simulink library "Decoders_Lib"  (R2023a)
settings: Solver=ode45  StartTime=0.0  StopTime=10.0  RelTol=1e-3  EnableMultiTasking=on
(part 1 of 2)
settings Model: Creator=uzivatel  LastModifiedBy=Jozko Mrkvicka
settings SolverCC: AlgebraicLoopSolver=TrustRegion
settings DataIOCC: LimitDataPoints=on  SaveFormat=Array  ReturnWorkspaceOutputs=off
settings OptimizationCC: LifeSpan=inf
settings DebuggingCC: UnderspecifiedInitializationDetection=Classic  MergeDetectMultiDrivingBlocksExec=none  SolverPrmCheckMsg=warning  UnconnectedInputMsg=warning  UnconnectedOutputMsg=warning  UnconnectedLineMsg=warning  StateNameClashWarn=warning  SFUnexpectedBacktrackingDiag=warning  SFNoUnconditionalDefaultTransitionDiag=warning  ArithmeticOperatorsInVariantConditions=warning
settings HardwareCC: ProdBitPerPointer=32  ProdBitPerSizeT=32  ProdBitPerPtrDiffT=32  ProdLargestAtomicFloat=None  ProdIntDivRoundTo=Undefined  ProdEndianess=Unspecified  ProdWordSize=32  ProdHWDeviceType=32-bit Generic
settings ModelReferenceCC: EnableRefExpFcnMdlSchedulingChecks=on  PropagateSignalLabelsOutOfModel=off
settings SFSimCC: SimUseLocalCustomCode=off  CustomCodeUndefinedFunction=UseInterfaceOnly
settings RTWCC: RTWUseLocalCustomCode=off
settings CodeAppCC: StateflowObjectComments=on
settings GRTTargetCC: TargetLangStandard=C89/C90 (ANSI)
settings ConfigComp: CovMetricSettings=dw  CovSaveCumulativeToWorkspaceVar=on  CovSaveSingleToWorkspaceVar=on  CovExternalEMLEnable=off

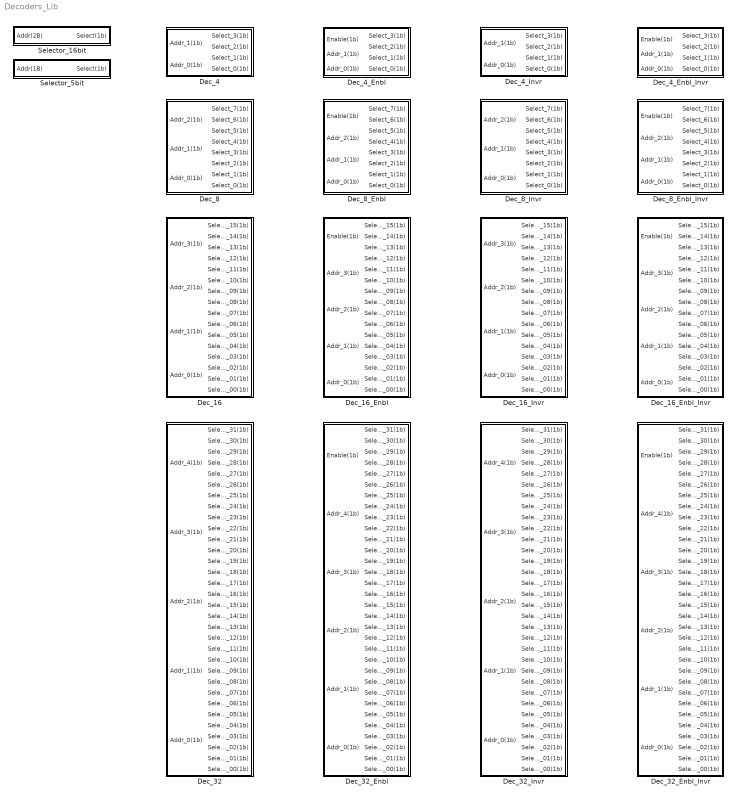
== system Decoders_Lib ==
  Dec_16 : Subsystem  TreatAsAtomicUnit=on
  Dec_16_Enbl : Subsystem  TreatAsAtomicUnit=on
  Dec_16_Enbl_Invr : Subsystem  TreatAsAtomicUnit=on
  Dec_16_Invr : Subsystem  TreatAsAtomicUnit=on
  Dec_32 : Subsystem  TreatAsAtomicUnit=on
  Dec_32_Enbl : Subsystem  TreatAsAtomicUnit=on
  Dec_32_Enbl_Invr : Subsystem  TreatAsAtomicUnit=on
  Dec_32_Invr : Subsystem  TreatAsAtomicUnit=on
  Dec_4 : Subsystem  TreatAsAtomicUnit=on
  Dec_4_Enbl : Subsystem  TreatAsAtomicUnit=on
  Dec_4_Enbl_Invr : Subsystem  TreatAsAtomicUnit=on
  Dec_4_Invr : Subsystem  TreatAsAtomicUnit=on
  Dec_8 : Subsystem  TreatAsAtomicUnit=on
  Dec_8_Enbl : Subsystem  TreatAsAtomicUnit=on
  Dec_8_Enbl_Invr : Subsystem  TreatAsAtomicUnit=on
  Dec_8_Invr : Subsystem  TreatAsAtomicUnit=on
  Selector_16bit : Subsystem
  Selector_5bit : Subsystem

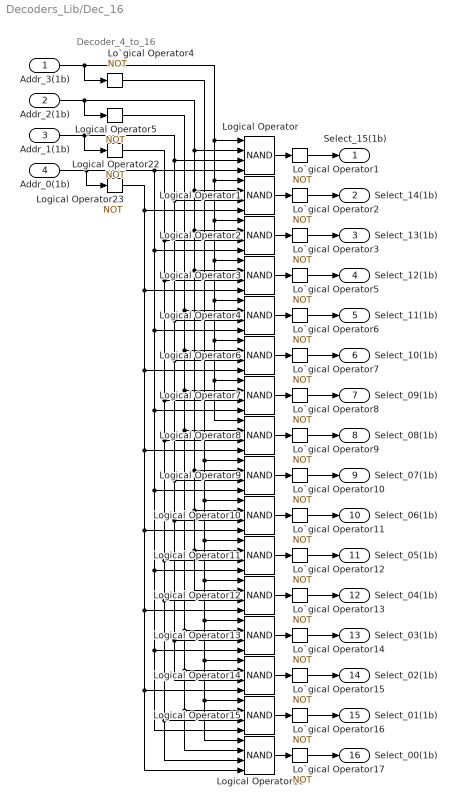
== system Decoders_Lib/Dec_16 ==
  note: Decoder_4_to_16
  Addr_3(1b) : Inport
  Addr_2(1b) : Inport  Port=2
  Addr_1(1b) : Inport  Port=3
  Addr_0(1b) : Inport  Port=4
  Lo`gical Operator{1..17} (17 alike) : Logic  Operator=NOT  IconShape=distinctive  AllPortsSameDT=off  OutDataTypeStr=boolean
  Logical Operator{,1..4,6..16} (16 alike) : Logic  Operator=NAND  Inputs=4  IconShape=distinctive  AllPortsSameDT=off  OutDataTypeStr=boolean
  Logical Operator22 : Logic  Operator=NOT  IconShape=distinctive  AllPortsSameDT=off  OutDataTypeStr=boolean
  Logical Operator23 : Logic  Operator=NOT  IconShape=distinctive  AllPortsSameDT=off  OutDataTypeStr=boolean
  Logical Operator5 : Logic  Operator=NOT  IconShape=distinctive  AllPortsSameDT=off  OutDataTypeStr=boolean
  Select_15(1b) : Outport
  Select_14(1b) : Outport  Port=2
  Select_13(1b) : Outport  Port=3
  Select_12(1b) : Outport  Port=4
  Select_11(1b) : Outport  Port=5
  Select_10(1b) : Outport  Port=6
  Select_09(1b) : Outport  Port=7
  Select_08(1b) : Outport  Port=8
  Select_07(1b) : Outport  Port=9
  Select_06(1b) : Outport  Port=10
  Select_05(1b) : Outport  Port=11
  Select_04(1b) : Outport  Port=12
  Select_03(1b) : Outport  Port=13
  Select_02(1b) : Outport  Port=14
  Select_01(1b) : Outport  Port=15
  Select_00(1b) : Outport  Port=16
  wires:
  Logical Operator22/1 -> Logical Operator2/3, Logical Operator3/3, Logical Operator15/3, Logical Operator16/3, Logical Operator12/3, Logical Operator11/3, Logical Operator8/3, Logical Operator7/3
  Addr_0(1b)/1 -> Logical Operator23/1, Logical Operator/4, Logical Operator9/4, Logical Operator11/4, Logical Operator15/4, Logical Operator13/4, Logical Operator7/4, Logical Operator4/4, Logical Operator2/4
  Logical Operator23/1 -> Logical Operator1/4, Logical Operator16/4, Logical Operator14/4, Logical Operator12/4, Logical Operator10/4, Logical Operator8/4, Logical Operator6/4, Logical Operator3/4
  Logical Operator5/1 -> Logical Operator16/2, Logical Operator15/2, Logical Operator14/2, Logical Operator13/2, Logical Operator8/2, Logical Operator7/2, Logical Operator6/2, Logical Operator4/2
  Addr_3(1b)/1 -> Lo`gical Operator4/1, Logical Operator8/1, Logical Operator7/1, Logical Operator6/1, Logical Operator4/1, Logical Operator3/1, Logical Operator2/1, Logical Operator1/1, Logical Operator/1
  Addr_1(1b)/1 -> Logical Operator22/1, Logical Operator14/3, Logical Operator13/3, Logical Operator10/3, Logical Operator9/3, Logical Operator6/3, Logical Operator4/3, Logical Operator1/3, Logical Operator/3
  Addr_2(1b)/1 -> Logical Operator5/1, Logical Operator3/2, Logical Operator9/2, Logical Operator12/2, Logical Operator11/2, Logical Operator10/2, Logical Operator2/2, Logical Operator1/2, Logical Operator/2
  Lo`gical Operator4/1 -> Logical Operator16/1, Logical Operator15/1, Logical Operator14/1, Logical Operator13/1, Logical Operator12/1, Logical Operator11/1, Logical Operator10/1, Logical Operator9/1
  Logical Operator16/1 -> Lo`gical Operator17/1
  Logical Operator15/1 -> Lo`gical Operator16/1
  Logical Operator14/1 -> Lo`gical Operator15/1
  Logical Operator13/1 -> Lo`gical Operator14/1
  Logical Operator12/1 -> Lo`gical Operator13/1
  Logical Operator11/1 -> Lo`gical Operator12/1
  Logical Operator10/1 -> Lo`gical Operator11/1
  Logical Operator9/1 -> Lo`gical Operator10/1
  Logical Operator8/1 -> Lo`gical Operator9/1
  Logical Operator7/1 -> Lo`gical Operator8/1
  Logical Operator6/1 -> Lo`gical Operator7/1
  Logical Operator4/1 -> Lo`gical Operator6/1
  Logical Operator1/1 -> Lo`gical Operator2/1
  Logical Operator2/1 -> Lo`gical Operator3/1
  Logical Operator3/1 -> Lo`gical Operator5/1
  Logical Operator/1 -> Lo`gical Operator1/1
  Lo`gical Operator1/1 -> Select_15(1b)/1
  Lo`gical Operator2/1 -> Select_14(1b)/1
  Lo`gical Operator3/1 -> Select_13(1b)/1
  Lo`gical Operator5/1 -> Select_12(1b)/1
  Lo`gical Operator6/1 -> Select_11(1b)/1
  Lo`gical Operator7/1 -> Select_10(1b)/1
  Lo`gical Operator8/1 -> Select_09(1b)/1
  Lo`gical Operator9/1 -> Select_08(1b)/1
  Lo`gical Operator10/1 -> Select_07(1b)/1
  Lo`gical Operator11/1 -> Select_06(1b)/1
  Lo`gical Operator12/1 -> Select_05(1b)/1
  Lo`gical Operator13/1 -> Select_04(1b)/1
  Lo`gical Operator14/1 -> Select_03(1b)/1
  Lo`gical Operator15/1 -> Select_02(1b)/1
  Lo`gical Operator16/1 -> Select_01(1b)/1
  Lo`gical Operator17/1 -> Select_00(1b)/1

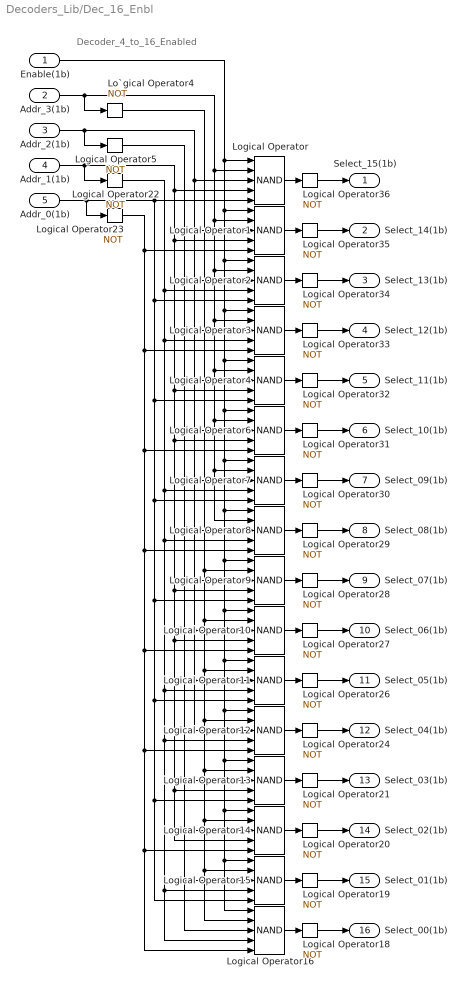
== system Decoders_Lib/Dec_16_Enbl ==
  note: Decoder_4_to_16_Enabled
  Enable(1b) : Inport
  Addr_3(1b) : Inport  Port=2
  Addr_2(1b) : Inport  Port=3
  Addr_1(1b) : Inport  Port=4
  Addr_0(1b) : Inport  Port=5
  Lo`gical Operator4 : Logic  Operator=NOT  IconShape=distinctive  AllPortsSameDT=off  OutDataTypeStr=boolean
  Logical Operator{,1..4,6..16} (16 alike) : Logic  Operator=NAND  Inputs=5  IconShape=distinctive  AllPortsSameDT=off  OutDataTypeStr=boolean
  Logical Operator{5,18..24,26..36} (19 alike) : Logic  Operator=NOT  IconShape=distinctive  AllPortsSameDT=off  OutDataTypeStr=boolean
  Select_15(1b) : Outport
  Select_14(1b) : Outport  Port=2
  Select_13(1b) : Outport  Port=3
  Select_12(1b) : Outport  Port=4
  Select_11(1b) : Outport  Port=5
  Select_10(1b) : Outport  Port=6
  Select_09(1b) : Outport  Port=7
  Select_08(1b) : Outport  Port=8
  Select_07(1b) : Outport  Port=9
  Select_06(1b) : Outport  Port=10
  Select_05(1b) : Outport  Port=11
  Select_04(1b) : Outport  Port=12
  Select_03(1b) : Outport  Port=13
  Select_02(1b) : Outport  Port=14
  Select_01(1b) : Outport  Port=15
  Select_00(1b) : Outport  Port=16
  wires:
  Logical Operator22/1 -> Logical Operator2/4, Logical Operator3/4, Logical Operator7/4, Logical Operator8/4, Logical Operator11/4, Logical Operator12/4, Logical Operator15/4, Logical Operator16/4
  Addr_0(1b)/1 -> Logical Operator/5, Logical Operator2/5, Logical Operator4/5, Logical Operator7/5, Logical Operator9/5, Logical Operator11/5, Logical Operator13/5, Logical Operator15/5, Logical Operator23/1
  Logical Operator23/1 -> Logical Operator1/5, Logical Operator3/5, Logical Operator6/5, Logical Operator8/5, Logical Operator10/5, Logical Operator12/5, Logical Operator14/5, Logical Operator16/5
  Logical Operator5/1 -> Logical Operator4/3, Logical Operator6/3, Logical Operator7/3, Logical Operator8/3, Logical Operator13/3, Logical Operator14/3, Logical Operator15/3, Logical Operator16/3
  Addr_3(1b)/1 -> Logical Operator/2, Logical Operator1/2, Logical Operator2/2, Logical Operator3/2, Logical Operator4/2, Logical Operator6/2, Logical Operator7/2, Logical Operator8/2, Lo`gical Operator4/1
  Addr_1(1b)/1 -> Logical Operator/4, Logical Operator1/4, Logical Operator4/4, Logical Operator6/4, Logical Operator9/4, Logical Operator10/4, Logical Operator13/4, Logical Operator14/4, Logical Operator22/1
  Addr_2(1b)/1 -> Logical Operator/3, Logical Operator1/3, Logical Operator2/3, Logical Operator3/3, Logical Operator9/3, Logical Operator10/3, Logical Operator11/3, Logical Operator12/3, Logical Operator5/1
  Lo`gical Operator4/1 -> Logical Operator9/2, Logical Operator10/2, Logical Operator11/2, Logical Operator12/2, Logical Operator13/2, Logical Operator14/2, Logical Operator15/2, Logical Operator16/2
  Logical Operator16/1 -> Logical Operator18/1
  Logical Operator15/1 -> Logical Operator19/1
  Logical Operator14/1 -> Logical Operator20/1
  Logical Operator13/1 -> Logical Operator21/1
  Logical Operator12/1 -> Logical Operator24/1
  Logical Operator11/1 -> Logical Operator26/1
  Logical Operator10/1 -> Logical Operator27/1
  Logical Operator9/1 -> Logical Operator28/1
  Logical Operator8/1 -> Logical Operator29/1
  Logical Operator7/1 -> Logical Operator30/1
  Logical Operator6/1 -> Logical Operator31/1
  Logical Operator4/1 -> Logical Operator32/1
  Logical Operator1/1 -> Logical Operator35/1
  Logical Operator2/1 -> Logical Operator34/1
  Logical Operator3/1 -> Logical Operator33/1
  Logical Operator/1 -> Logical Operator36/1
  Enable(1b)/1 -> Logical Operator/1, Logical Operator1/1, Logical Operator2/1, Logical Operator3/1, Logical Operator4/1, Logical Operator6/1, Logical Operator7/1, Logical Operator8/1, Logical Operator9/1, Logical Operator10/1, Logical Operator11/1, Logical Operator12/1, Logical Operator13/1, Logical Operator14/1, Logical Operator15/1, Logical Operator16/1
  Logical Operator18/1 -> Select_00(1b)/1
  Logical Operator19/1 -> Select_01(1b)/1
  Logical Operator20/1 -> Select_02(1b)/1
  Logical Operator21/1 -> Select_03(1b)/1
  Logical Operator24/1 -> Select_04(1b)/1
  Logical Operator26/1 -> Select_05(1b)/1
  Logical Operator27/1 -> Select_06(1b)/1
  Logical Operator28/1 -> Select_07(1b)/1
  Logical Operator29/1 -> Select_08(1b)/1
  Logical Operator30/1 -> Select_09(1b)/1
  Logical Operator31/1 -> Select_10(1b)/1
  Logical Operator32/1 -> Select_11(1b)/1
  Logical Operator33/1 -> Select_12(1b)/1
  Logical Operator34/1 -> Select_13(1b)/1
  Logical Operator35/1 -> Select_14(1b)/1
  Logical Operator36/1 -> Select_15(1b)/1

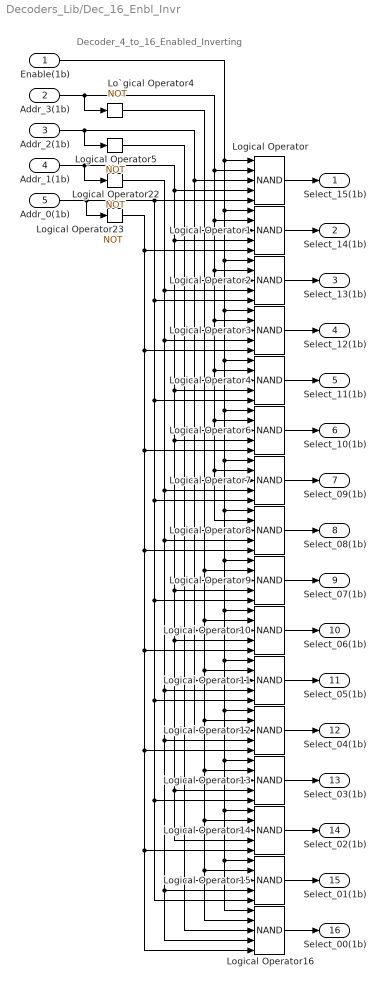
== system Decoders_Lib/Dec_16_Enbl_Invr ==
  note: Decoder_4_to_16_Enabled_Inverting
  Enable(1b) : Inport
  Addr_3(1b) : Inport  Port=2
  Addr_2(1b) : Inport  Port=3
  Addr_1(1b) : Inport  Port=4
  Addr_0(1b) : Inport  Port=5
  Lo`gical Operator4 : Logic  Operator=NOT  IconShape=distinctive  AllPortsSameDT=off  OutDataTypeStr=boolean
  Logical Operator{,1..4,6..16} (16 alike) : Logic  Operator=NAND  Inputs=5  IconShape=distinctive  AllPortsSameDT=off  OutDataTypeStr=boolean
  Logical Operator22 : Logic  Operator=NOT  IconShape=distinctive  AllPortsSameDT=off  OutDataTypeStr=boolean
  Logical Operator23 : Logic  Operator=NOT  IconShape=distinctive  AllPortsSameDT=off  OutDataTypeStr=boolean
  Logical Operator5 : Logic  Operator=NOT  IconShape=distinctive  AllPortsSameDT=off  OutDataTypeStr=boolean
  Select_15(1b) : Outport
  Select_14(1b) : Outport  Port=2
  Select_13(1b) : Outport  Port=3
  Select_12(1b) : Outport  Port=4
  Select_11(1b) : Outport  Port=5
  Select_10(1b) : Outport  Port=6
  Select_09(1b) : Outport  Port=7
  Select_08(1b) : Outport  Port=8
  Select_07(1b) : Outport  Port=9
  Select_06(1b) : Outport  Port=10
  Select_05(1b) : Outport  Port=11
  Select_04(1b) : Outport  Port=12
  Select_03(1b) : Outport  Port=13
  Select_02(1b) : Outport  Port=14
  Select_01(1b) : Outport  Port=15
  Select_00(1b) : Outport  Port=16
  wires:
  Logical Operator22/1 -> Logical Operator2/4, Logical Operator3/4, Logical Operator7/4, Logical Operator8/4, Logical Operator11/4, Logical Operator12/4, Logical Operator15/4, Logical Operator16/4
  Addr_0(1b)/1 -> Logical Operator/5, Logical Operator2/5, Logical Operator4/5, Logical Operator7/5, Logical Operator9/5, Logical Operator11/5, Logical Operator13/5, Logical Operator15/5, Logical Operator23/1
  Logical Operator23/1 -> Logical Operator1/5, Logical Operator3/5, Logical Operator6/5, Logical Operator8/5, Logical Operator10/5, Logical Operator12/5, Logical Operator14/5, Logical Operator16/5
  Logical Operator5/1 -> Logical Operator4/3, Logical Operator6/3, Logical Operator7/3, Logical Operator8/3, Logical Operator13/3, Logical Operator14/3, Logical Operator15/3, Logical Operator16/3
  Addr_3(1b)/1 -> Logical Operator/2, Logical Operator1/2, Logical Operator2/2, Logical Operator3/2, Logical Operator4/2, Logical Operator6/2, Logical Operator7/2, Logical Operator8/2, Lo`gical Operator4/1
  Addr_1(1b)/1 -> Logical Operator/4, Logical Operator1/4, Logical Operator4/4, Logical Operator6/4, Logical Operator9/4, Logical Operator10/4, Logical Operator13/4, Logical Operator14/4, Logical Operator22/1
  Addr_2(1b)/1 -> Logical Operator/3, Logical Operator1/3, Logical Operator2/3, Logical Operator3/3, Logical Operator9/3, Logical Operator10/3, Logical Operator11/3, Logical Operator12/3, Logical Operator5/1
  Lo`gical Operator4/1 -> Logical Operator9/2, Logical Operator10/2, Logical Operator11/2, Logical Operator12/2, Logical Operator13/2, Logical Operator14/2, Logical Operator15/2, Logical Operator16/2
  Logical Operator16/1 -> Select_00(1b)/1
  Logical Operator15/1 -> Select_01(1b)/1
  Logical Operator14/1 -> Select_02(1b)/1
  Logical Operator13/1 -> Select_03(1b)/1
  Logical Operator12/1 -> Select_04(1b)/1
  Logical Operator11/1 -> Select_05(1b)/1
  Logical Operator10/1 -> Select_06(1b)/1
  Logical Operator9/1 -> Select_07(1b)/1
  Logical Operator8/1 -> Select_08(1b)/1
  Logical Operator7/1 -> Select_09(1b)/1
  Logical Operator6/1 -> Select_10(1b)/1
  Logical Operator4/1 -> Select_11(1b)/1
  Logical Operator1/1 -> Select_14(1b)/1
  Logical Operator2/1 -> Select_13(1b)/1
  Logical Operator3/1 -> Select_12(1b)/1
  Logical Operator/1 -> Select_15(1b)/1
  Enable(1b)/1 -> Logical Operator/1, Logical Operator1/1, Logical Operator2/1, Logical Operator3/1, Logical Operator4/1, Logical Operator6/1, Logical Operator7/1, Logical Operator8/1, Logical Operator9/1, Logical Operator10/1, Logical Operator11/1, Logical Operator12/1, Logical Operator13/1, Logical Operator14/1, Logical Operator15/1, Logical Operator16/1

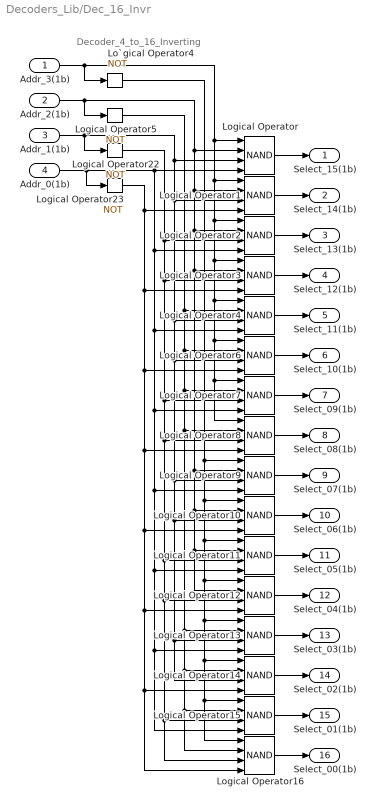
== system Decoders_Lib/Dec_16_Invr ==
  note: Decoder_4_to_16_Inverting
  Addr_3(1b) : Inport
  Addr_2(1b) : Inport  Port=2
  Addr_1(1b) : Inport  Port=3
  Addr_0(1b) : Inport  Port=4
  Lo`gical Operator4 : Logic  Operator=NOT  IconShape=distinctive  AllPortsSameDT=off  OutDataTypeStr=boolean
  Logical Operator{,1..4,6..16} (16 alike) : Logic  Operator=NAND  Inputs=4  IconShape=distinctive  AllPortsSameDT=off  OutDataTypeStr=boolean
  Logical Operator22 : Logic  Operator=NOT  IconShape=distinctive  AllPortsSameDT=off  OutDataTypeStr=boolean
  Logical Operator23 : Logic  Operator=NOT  IconShape=distinctive  AllPortsSameDT=off  OutDataTypeStr=boolean
  Logical Operator5 : Logic  Operator=NOT  IconShape=distinctive  AllPortsSameDT=off  OutDataTypeStr=boolean
  Select_15(1b) : Outport
  Select_14(1b) : Outport  Port=2
  Select_13(1b) : Outport  Port=3
  Select_12(1b) : Outport  Port=4
  Select_11(1b) : Outport  Port=5
  Select_10(1b) : Outport  Port=6
  Select_09(1b) : Outport  Port=7
  Select_08(1b) : Outport  Port=8
  Select_07(1b) : Outport  Port=9
  Select_06(1b) : Outport  Port=10
  Select_05(1b) : Outport  Port=11
  Select_04(1b) : Outport  Port=12
  Select_03(1b) : Outport  Port=13
  Select_02(1b) : Outport  Port=14
  Select_01(1b) : Outport  Port=15
  Select_00(1b) : Outport  Port=16
  wires:
  Logical Operator22/1 -> Logical Operator2/3, Logical Operator3/3, Logical Operator15/3, Logical Operator16/3, Logical Operator12/3, Logical Operator11/3, Logical Operator8/3, Logical Operator7/3
  Addr_0(1b)/1 -> Logical Operator23/1, Logical Operator/4, Logical Operator9/4, Logical Operator11/4, Logical Operator15/4, Logical Operator13/4, Logical Operator7/4, Logical Operator4/4, Logical Operator2/4
  Logical Operator23/1 -> Logical Operator1/4, Logical Operator16/4, Logical Operator14/4, Logical Operator12/4, Logical Operator10/4, Logical Operator8/4, Logical Operator6/4, Logical Operator3/4
  Logical Operator5/1 -> Logical Operator16/2, Logical Operator15/2, Logical Operator14/2, Logical Operator13/2, Logical Operator8/2, Logical Operator7/2, Logical Operator6/2, Logical Operator4/2
  Addr_3(1b)/1 -> Lo`gical Operator4/1, Logical Operator8/1, Logical Operator7/1, Logical Operator6/1, Logical Operator4/1, Logical Operator3/1, Logical Operator2/1, Logical Operator1/1, Logical Operator/1
  Addr_1(1b)/1 -> Logical Operator22/1, Logical Operator14/3, Logical Operator13/3, Logical Operator10/3, Logical Operator9/3, Logical Operator6/3, Logical Operator4/3, Logical Operator1/3, Logical Operator/3
  Addr_2(1b)/1 -> Logical Operator5/1, Logical Operator3/2, Logical Operator9/2, Logical Operator12/2, Logical Operator11/2, Logical Operator10/2, Logical Operator2/2, Logical Operator1/2, Logical Operator/2
  Lo`gical Operator4/1 -> Logical Operator16/1, Logical Operator15/1, Logical Operator14/1, Logical Operator13/1, Logical Operator12/1, Logical Operator11/1, Logical Operator10/1, Logical Operator9/1
  Logical Operator16/1 -> Select_00(1b)/1
  Logical Operator15/1 -> Select_01(1b)/1
  Logical Operator14/1 -> Select_02(1b)/1
  Logical Operator13/1 -> Select_03(1b)/1
  Logical Operator12/1 -> Select_04(1b)/1
  Logical Operator11/1 -> Select_05(1b)/1
  Logical Operator10/1 -> Select_06(1b)/1
  Logical Operator9/1 -> Select_07(1b)/1
  Logical Operator8/1 -> Select_08(1b)/1
  Logical Operator7/1 -> Select_09(1b)/1
  Logical Operator6/1 -> Select_10(1b)/1
  Logical Operator4/1 -> Select_11(1b)/1
  Logical Operator1/1 -> Select_14(1b)/1
  Logical Operator2/1 -> Select_13(1b)/1
  Logical Operator3/1 -> Select_12(1b)/1
  Logical Operator/1 -> Select_15(1b)/1

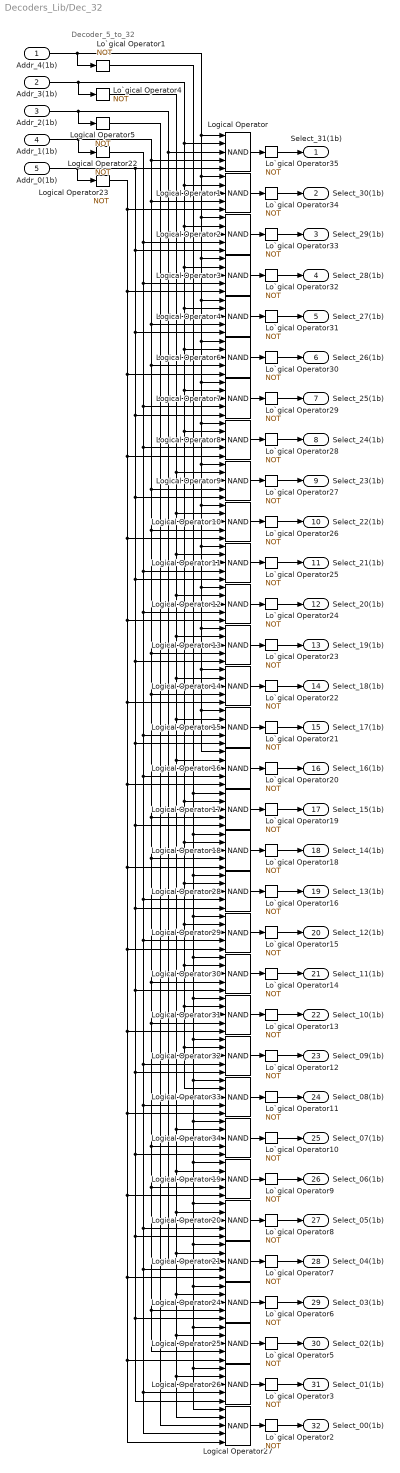
== system Decoders_Lib/Dec_32 ==
  note: Decoder_5_to_32
  Addr_4(1b) : Inport
  Addr_3(1b) : Inport  Port=2
  Addr_2(1b) : Inport  Port=3
  Addr_1(1b) : Inport  Port=4
  Addr_0(1b) : Inport  Port=5
  Lo`gical Operator{1..16,18..35} (34 alike) : Logic  Operator=NOT  IconShape=distinctive  AllPortsSameDT=off  OutDataTypeStr=boolean
  Logical Operator{,1..4,6..21,24..34} (32 alike) : Logic  Operator=NAND  Inputs=5  IconShape=distinctive  AllPortsSameDT=off  OutDataTypeStr=boolean
  Logical Operator22 : Logic  Operator=NOT  IconShape=distinctive  AllPortsSameDT=off  OutDataTypeStr=boolean
  Logical Operator23 : Logic  Operator=NOT  IconShape=distinctive  AllPortsSameDT=off  OutDataTypeStr=boolean
  Logical Operator5 : Logic  Operator=NOT  IconShape=distinctive  AllPortsSameDT=off  OutDataTypeStr=boolean
  Select_31(1b) : Outport
  Select_30(1b) : Outport  Port=2
  Select_29(1b) : Outport  Port=3
  Select_28(1b) : Outport  Port=4
  Select_27(1b) : Outport  Port=5
  Select_26(1b) : Outport  Port=6
  Select_25(1b) : Outport  Port=7
  Select_24(1b) : Outport  Port=8
  Select_23(1b) : Outport  Port=9
  Select_22(1b) : Outport  Port=10
  Select_21(1b) : Outport  Port=11
  Select_20(1b) : Outport  Port=12
  Select_19(1b) : Outport  Port=13
  Select_18(1b) : Outport  Port=14
  Select_17(1b) : Outport  Port=15
  Select_16(1b) : Outport  Port=16
  Select_15(1b) : Outport  Port=17
  Select_14(1b) : Outport  Port=18
  Select_13(1b) : Outport  Port=19
  Select_12(1b) : Outport  Port=20
  Select_11(1b) : Outport  Port=21
  Select_10(1b) : Outport  Port=22
  Select_09(1b) : Outport  Port=23
  Select_08(1b) : Outport  Port=24
  Select_07(1b) : Outport  Port=25
  Select_06(1b) : Outport  Port=26
  Select_05(1b) : Outport  Port=27
  Select_04(1b) : Outport  Port=28
  Select_03(1b) : Outport  Port=29
  Select_02(1b) : Outport  Port=30
  Select_01(1b) : Outport  Port=31
  Select_00(1b) : Outport  Port=32
  wires:
  Logical Operator16/1 -> Lo`gical Operator20/1
  Logical Operator15/1 -> Lo`gical Operator21/1
  Logical Operator14/1 -> Lo`gical Operator22/1
  Logical Operator13/1 -> Lo`gical Operator23/1
  Logical Operator12/1 -> Lo`gical Operator24/1
  Logical Operator11/1 -> Lo`gical Operator25/1
  Logical Operator10/1 -> Lo`gical Operator26/1
  Logical Operator9/1 -> Lo`gical Operator27/1
  Logical Operator8/1 -> Lo`gical Operator28/1
  Logical Operator7/1 -> Lo`gical Operator29/1
  Logical Operator6/1 -> Lo`gical Operator30/1
  Logical Operator4/1 -> Lo`gical Operator31/1
  Logical Operator1/1 -> Lo`gical Operator34/1
  Logical Operator2/1 -> Lo`gical Operator33/1
  Logical Operator3/1 -> Lo`gical Operator32/1
  Logical Operator/1 -> Lo`gical Operator35/1
  Logical Operator22/1 -> Logical Operator27/4, Logical Operator26/4, Logical Operator21/4, Logical Operator20/4, Logical Operator33/4, Logical Operator32/4, Logical Operator29/4, Logical Operator28/4, Logical Operator16/4, Logical Operator15/4, Logical Operator12/4, Logical Operator11/4, Logical Operator8/4, Logical Operator7/4, Logical Operator3/4, Logical Operator2/4
  Addr_0(1b)/1 -> Logical Operator26/5, Logical Operator24/5, Logical Operator20/5, Logical Operator34/5, Logical Operator32/5, Logical Operator30/5, Logical Operator28/5, Logical Operator17/5, Logical Operator15/5, Logical Operator13/5, Logical Operator11/5, Logical Operator9/5, Logical Operator7/5, Logical Operator4/5, Logical Operator2/5, Logical Operator/5, Logical Operator23/1
  Logical Operator23/1 -> Logical Operator27/5, Logical Operator25/5, Logical Operator21/5, Logical Operator19/5, Logical Operator33/5, Logical Operator31/5, Logical Operator29/5, Logical Operator18/5, Logical Operator16/5, Logical Operator14/5, Logical Operator12/5, Logical Operator10/5, Logical Operator8/5, Logical Operator6/5, Logical Operator3/5, Logical Operator1/5
  Logical Operator5/1 -> Logical Operator27/3, Logical Operator26/3, Logical Operator25/3, Logical Operator24/3, Logical Operator33/3, Logical Operator32/3, Logical Operator31/3, Logical Operator30/3, Logical Operator16/3, Logical Operator15/3, Logical Operator14/3, Logical Operator13/3, Logical Operator8/3, Logical Operator7/3, Logical Operator6/3, Logical Operator4/3
  Addr_3(1b)/1 -> Lo`gical Operator4/1, Logical Operator33/2, Logical Operator32/2, Logical Operator31/2, Logical Operator30/2, Logical Operator29/2, Logical Operator28/2, Logical Operator18/2, Logical Operator17/2, Logical Operator8/2, Logical Operator7/2, Logical Operator6/2, Logical Operator4/2, Logical Operator3/2, Logical Operator2/2, Logical Operator1/2, Logical Operator/2
  Addr_1(1b)/1 -> Logical Operator22/1, Logical Operator25/4, Logical Operator24/4, Logical Operator19/4, Logical Operator34/4, Logical Operator31/4, Logical Operator30/4, Logical Operator18/4, Logical Operator17/4, Logical Operator14/4, Logical Operator13/4, Logical Operator10/4, Logical Operator9/4, Logical Operator6/4, Logical Operator4/4, Logical Operator1/4, Logical Operator/4
  Addr_2(1b)/1 -> Logical Operator21/3, Logical Operator20/3, Logical Operator19/3, Logical Operator34/3, Logical Operator29/3, Logical Operator28/3, Logical Operator18/3, Logical Operator17/3, Logical Operator12/3, Logical Operator11/3, Logical Operator10/3, Logical Operator9/3, Logical Operator3/3, Logical Operator2/3, Logical Operator1/3, Logical Operator/3, Logical Operator5/1
  Lo`gical Operator4/1 -> Logical Operator27/2, Logical Operator26/2, Logical Operator25/2, Logical Operator24/2, Logical Operator21/2, Logical Operator20/2, Logical Operator19/2, Logical Operator34/2, Logical Operator16/2, Logical Operator15/2, Logical Operator14/2, Logical Operator13/2, Logical Operator12/2, Logical Operator11/2, Logical Operator10/2, Logical Operator9/2
  Logical Operator27/1 -> Lo`gical Operator2/1
  Logical Operator26/1 -> Lo`gical Operator3/1
  Logical Operator25/1 -> Lo`gical Operator5/1
  Logical Operator24/1 -> Lo`gical Operator6/1
  Logical Operator21/1 -> Lo`gical Operator7/1
  Logical Operator20/1 -> Lo`gical Operator8/1
  Logical Operator19/1 -> Lo`gical Operator9/1
  Logical Operator34/1 -> Lo`gical Operator10/1
  Logical Operator33/1 -> Lo`gical Operator11/1
  Logical Operator32/1 -> Lo`gical Operator12/1
  Logical Operator31/1 -> Lo`gical Operator13/1
  Logical Operator30/1 -> Lo`gical Operator14/1
  Logical Operator18/1 -> Lo`gical Operator18/1
  Logical Operator28/1 -> Lo`gical Operator16/1
  Logical Operator29/1 -> Lo`gical Operator15/1
  Logical Operator17/1 -> Lo`gical Operator19/1
  Lo`gical Operator1/1 -> Logical Operator27/1, Logical Operator26/1, Logical Operator25/1, Logical Operator24/1, Logical Operator21/1, Logical Operator20/1, Logical Operator19/1, Logical Operator34/1, Logical Operator33/1, Logical Operator32/1, Logical Operator31/1, Logical Operator30/1, Logical Operator29/1, Logical Operator28/1, Logical Operator18/1, Logical Operator17/1
  Addr_4(1b)/1 -> Logical Operator16/1, Logical Operator15/1, Logical Operator14/1, Logical Operator13/1, Logical Operator12/1, Logical Operator11/1, Logical Operator10/1, Logical Operator9/1, Logical Operator8/1, Logical Operator7/1, Logical Operator6/1, Logical Operator4/1, Logical Operator3/1, Logical Operator2/1, Logical Operator1/1, Logical Operator/1, Lo`gical Operator1/1
  Lo`gical Operator35/1 -> Select_31(1b)/1
  Lo`gical Operator34/1 -> Select_30(1b)/1
  Lo`gical Operator33/1 -> Select_29(1b)/1
  Lo`gical Operator32/1 -> Select_28(1b)/1
  Lo`gical Operator31/1 -> Select_27(1b)/1
  Lo`gical Operator30/1 -> Select_26(1b)/1
  Lo`gical Operator29/1 -> Select_25(1b)/1
  Lo`gical Operator28/1 -> Select_24(1b)/1
  Lo`gical Operator27/1 -> Select_23(1b)/1
  Lo`gical Operator26/1 -> Select_22(1b)/1
  Lo`gical Operator25/1 -> Select_21(1b)/1
  Lo`gical Operator24/1 -> Select_20(1b)/1
  Lo`gical Operator23/1 -> Select_19(1b)/1
  Lo`gical Operator22/1 -> Select_18(1b)/1
  Lo`gical Operator21/1 -> Select_17(1b)/1
  Lo`gical Operator20/1 -> Select_16(1b)/1
  Lo`gical Operator19/1 -> Select_15(1b)/1
  Lo`gical Operator18/1 -> Select_14(1b)/1
  Lo`gical Operator16/1 -> Select_13(1b)/1
  Lo`gical Operator15/1 -> Select_12(1b)/1
  Lo`gical Operator14/1 -> Select_11(1b)/1
  Lo`gical Operator13/1 -> Select_10(1b)/1
  Lo`gical Operator12/1 -> Select_09(1b)/1
  Lo`gical Operator11/1 -> Select_08(1b)/1
  Lo`gical Operator10/1 -> Select_07(1b)/1
  Lo`gical Operator9/1 -> Select_06(1b)/1
  Lo`gical Operator8/1 -> Select_05(1b)/1
  Lo`gical Operator7/1 -> Select_04(1b)/1
  Lo`gical Operator6/1 -> Select_03(1b)/1
  Lo`gical Operator5/1 -> Select_02(1b)/1
  Lo`gical Operator3/1 -> Select_01(1b)/1
  Lo`gical Operator2/1 -> Select_00(1b)/1

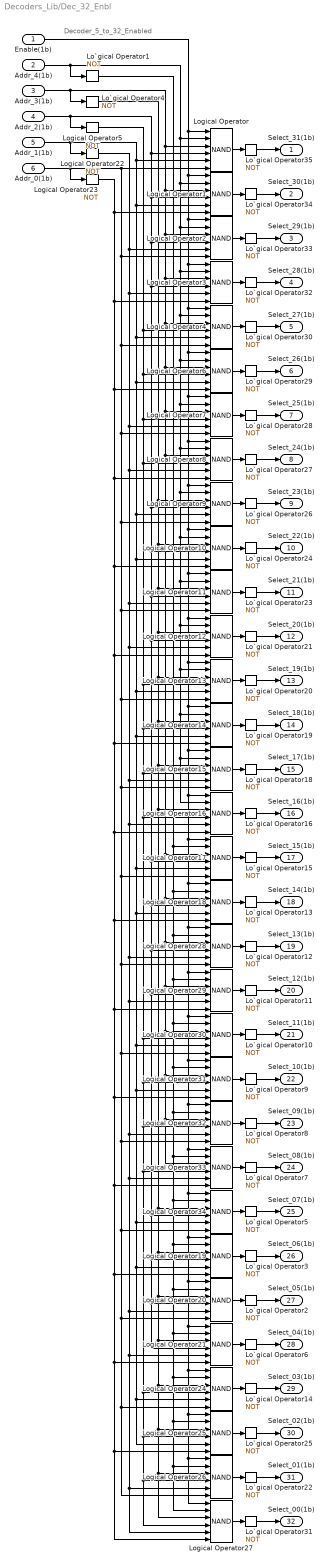
== system Decoders_Lib/Dec_32_Enbl ==
  note: Decoder_5_to_32_Enabled
  Enable(1b) : Inport
  Addr_4(1b) : Inport  Port=2
  Addr_3(1b) : Inport  Port=3
  Addr_2(1b) : Inport  Port=4
  Addr_1(1b) : Inport  Port=5
  Addr_0(1b) : Inport  Port=6
  Lo`gical Operator{1..16,18..35} (34 alike) : Logic  Operator=NOT  IconShape=distinctive  AllPortsSameDT=off  OutDataTypeStr=boolean
  Logical Operator{,1..4,6..21,24..34} (32 alike) : Logic  Operator=NAND  Inputs=6  IconShape=distinctive  AllPortsSameDT=off  OutDataTypeStr=boolean
  Logical Operator22 : Logic  Operator=NOT  IconShape=distinctive  AllPortsSameDT=off  OutDataTypeStr=boolean
  Logical Operator23 : Logic  Operator=NOT  IconShape=distinctive  AllPortsSameDT=off  OutDataTypeStr=boolean
  Logical Operator5 : Logic  Operator=NOT  IconShape=distinctive  AllPortsSameDT=off  OutDataTypeStr=boolean
  Select_31(1b) : Outport
  Select_30(1b) : Outport  Port=2
  Select_29(1b) : Outport  Port=3
  Select_28(1b) : Outport  Port=4
  Select_27(1b) : Outport  Port=5
  Select_26(1b) : Outport  Port=6
  Select_25(1b) : Outport  Port=7
  Select_24(1b) : Outport  Port=8
  Select_23(1b) : Outport  Port=9
  Select_22(1b) : Outport  Port=10
  Select_21(1b) : Outport  Port=11
  Select_20(1b) : Outport  Port=12
  Select_19(1b) : Outport  Port=13
  Select_18(1b) : Outport  Port=14
  Select_17(1b) : Outport  Port=15
  Select_16(1b) : Outport  Port=16
  Select_15(1b) : Outport  Port=17
  Select_14(1b) : Outport  Port=18
  Select_13(1b) : Outport  Port=19
  Select_12(1b) : Outport  Port=20
  Select_11(1b) : Outport  Port=21
  Select_10(1b) : Outport  Port=22
  Select_09(1b) : Outport  Port=23
  Select_08(1b) : Outport  Port=24
  Select_07(1b) : Outport  Port=25
  Select_06(1b) : Outport  Port=26
  Select_05(1b) : Outport  Port=27
  Select_04(1b) : Outport  Port=28
  Select_03(1b) : Outport  Port=29
  Select_02(1b) : Outport  Port=30
  Select_01(1b) : Outport  Port=31
  Select_00(1b) : Outport  Port=32
  wires:
  Logical Operator22/1 -> Logical Operator2/5, Logical Operator3/5, Logical Operator7/5, Logical Operator8/5, Logical Operator11/5, Logical Operator12/5, Logical Operator15/5, Logical Operator16/5, Logical Operator28/5, Logical Operator29/5, Logical Operator32/5, Logical Operator33/5, Logical Operator20/5, Logical Operator21/5, Logical Operator27/5, Logical Operator26/5
  Addr_0(1b)/1 -> Logical Operator2/6, Logical Operator4/6, Logical Operator7/6, Logical Operator9/6, Logical Operator11/6, Logical Operator13/6, Logical Operator15/6, Logical Operator17/6, Logical Operator28/6, Logical Operator30/6, Logical Operator32/6, Logical Operator34/6, Logical Operator20/6, Logical Operator24/6, Logical Operator26/6, Logical Operator/6, Logical Operator23/1
  Logical Operator23/1 -> Logical Operator1/6, Logical Operator3/6, Logical Operator6/6, Logical Operator8/6, Logical Operator10/6, Logical Operator12/6, Logical Operator14/6, Logical Operator16/6, Logical Operator18/6, Logical Operator29/6, Logical Operator31/6, Logical Operator33/6, Logical Operator19/6, Logical Operator21/6, Logical Operator27/6, Logical Operator25/6
  Logical Operator5/1 -> Logical Operator4/4, Logical Operator6/4, Logical Operator7/4, Logical Operator8/4, Logical Operator13/4, Logical Operator14/4, Logical Operator15/4, Logical Operator16/4, Logical Operator30/4, Logical Operator31/4, Logical Operator32/4, Logical Operator33/4, Logical Operator24/4, Logical Operator25/4, Logical Operator27/4, Logical Operator26/4
  Addr_3(1b)/1 -> Lo`gical Operator4/1, Logical Operator/3, Logical Operator1/3, Logical Operator2/3, Logical Operator3/3, Logical Operator4/3, Logical Operator6/3, Logical Operator7/3, Logical Operator8/3, Logical Operator17/3, Logical Operator18/3, Logical Operator28/3, Logical Operator29/3, Logical Operator30/3, Logical Operator31/3, Logical Operator33/3, Logical Operator32/3
  Addr_1(1b)/1 -> Logical Operator22/1, Logical Operator/5, Logical Operator1/5, Logical Operator4/5, Logical Operator6/5, Logical Operator9/5, Logical Operator10/5, Logical Operator13/5, Logical Operator14/5, Logical Operator17/5, Logical Operator18/5, Logical Operator30/5, Logical Operator31/5, Logical Operator34/5, Logical Operator19/5, Logical Operator24/5, Logical Operator25/5
  Addr_2(1b)/1 -> Logical Operator/4, Logical Operator1/4, Logical Operator2/4, Logical Operator3/4, Logical Operator9/4, Logical Operator10/4, Logical Operator11/4, Logical Operator12/4, Logical Operator17/4, Logical Operator18/4, Logical Operator28/4, Logical Operator29/4, Logical Operator34/4, Logical Operator19/4, Logical Operator21/4, Logical Operator20/4, Logical Operator5/1
  Lo`gical Operator4/1 -> Logical Operator9/3, Logical Operator10/3, Logical Operator11/3, Logical Operator12/3, Logical Operator13/3, Logical Operator14/3, Logical Operator15/3, Logical Operator16/3, Logical Operator34/3, Logical Operator19/3, Logical Operator20/3, Logical Operator21/3, Logical Operator24/3, Logical Operator25/3, Logical Operator26/3, Logical Operator27/3
  Lo`gical Operator1/1 -> Logical Operator17/2, Logical Operator18/2, Logical Operator28/2, Logical Operator29/2, Logical Operator30/2, Logical Operator31/2, Logical Operator32/2, Logical Operator33/2, Logical Operator34/2, Logical Operator19/2, Logical Operator20/2, Logical Operator21/2, Logical Operator24/2, Logical Operator25/2, Logical Operator26/2, Logical Operator27/2
  Addr_4(1b)/1 -> Logical Operator/2, Logical Operator1/2, Logical Operator2/2, Logical Operator3/2, Logical Operator4/2, Logical Operator6/2, Logical Operator7/2, Logical Operator8/2, Logical Operator9/2, Logical Operator10/2, Logical Operator11/2, Logical Operator12/2, Logical Operator13/2, Logical Operator14/2, Logical Operator15/2, Logical Operator16/2, Lo`gical Operator1/1
  Logical Operator3/1 -> Lo`gical Operator32/1
  Logical Operator4/1 -> Lo`gical Operator30/1
  Logical Operator7/1 -> Lo`gical Operator28/1
  Logical Operator16/1 -> Lo`gical Operator16/1
  Logical Operator8/1 -> Lo`gical Operator27/1
  Logical Operator15/1 -> Lo`gical Operator18/1
  Logical Operator14/1 -> Lo`gical Operator19/1
  Logical Operator11/1 -> Lo`gical Operator23/1
  Logical Operator12/1 -> Lo`gical Operator21/1
  Logical Operator9/1 -> Lo`gical Operator26/1
  Logical Operator34/1 -> Lo`gical Operator5/1
  Logical Operator30/1 -> Lo`gical Operator10/1
  Logical Operator10/1 -> Lo`gical Operator24/1
  Logical Operator31/1 -> Lo`gical Operator9/1
  Logical Operator29/1 -> Lo`gical Operator11/1
  Logical Operator24/1 -> Lo`gical Operator14/1
  Logical Operator1/1 -> Lo`gical Operator34/1
  Logical Operator18/1 -> Lo`gical Operator13/1
  Logical Operator28/1 -> Lo`gical Operator12/1
  Logical Operator33/1 -> Lo`gical Operator7/1
  Logical Operator6/1 -> Lo`gical Operator29/1
  Logical Operator19/1 -> Lo`gical Operator3/1
  Logical Operator26/1 -> Lo`gical Operator22/1
  Logical Operator20/1 -> Lo`gical Operator2/1
  Logical Operator32/1 -> Lo`gical Operator8/1
  Logical Operator2/1 -> Lo`gical Operator33/1
  Logical Operator21/1 -> Lo`gical Operator6/1
  Logical Operator13/1 -> Lo`gical Operator20/1
  Logical Operator17/1 -> Lo`gical Operator15/1
  Logical Operator27/1 -> Lo`gical Operator31/1
  Logical Operator25/1 -> Lo`gical Operator25/1
  Enable(1b)/1 -> Logical Operator/1, Logical Operator1/1, Logical Operator2/1, Logical Operator3/1, Logical Operator4/1, Logical Operator6/1, Logical Operator7/1, Logical Operator8/1, Logical Operator9/1, Logical Operator10/1, Logical Operator11/1, Logical Operator12/1, Logical Operator13/1, Logical Operator14/1, Logical Operator15/1, Logical Operator16/1, Logical Operator17/1, Logical Operator18/1, Logical Operator28/1, Logical Operator29/1, Logical Operator30/1, Logical Operator31/1, Logical Operator32/1, Logical Operator33/1, Logical Operator34/1, Logical Operator19/1, Logical Operator20/1, Logical Operator21/1, Logical Operator24/1, Logical Operator25/1, Logical Operator26/1, Logical Operator27/1
  Logical Operator/1 -> Lo`gical Operator35/1
  Lo`gical Operator35/1 -> Select_31(1b)/1
  Lo`gical Operator34/1 -> Select_30(1b)/1
  Lo`gical Operator33/1 -> Select_29(1b)/1
  Lo`gical Operator32/1 -> Select_28(1b)/1
  Lo`gical Operator30/1 -> Select_27(1b)/1
  Lo`gical Operator29/1 -> Select_26(1b)/1
  Lo`gical Operator28/1 -> Select_25(1b)/1
  Lo`gical Operator27/1 -> Select_24(1b)/1
  Lo`gical Operator26/1 -> Select_23(1b)/1
  Lo`gical Operator23/1 -> Select_21(1b)/1
  Lo`gical Operator10/1 -> Select_11(1b)/1
  Lo`gical Operator9/1 -> Select_10(1b)/1
  Lo`gical Operator8/1 -> Select_09(1b)/1
  Lo`gical Operator7/1 -> Select_08(1b)/1
  Lo`gical Operator11/1 -> Select_12(1b)/1
  Lo`gical Operator12/1 -> Select_13(1b)/1
  Lo`gical Operator13/1 -> Select_14(1b)/1
  Lo`gical Operator15/1 -> Select_15(1b)/1
  Lo`gical Operator18/1 -> Select_17(1b)/1
  Lo`gical Operator5/1 -> Select_07(1b)/1
  Lo`gical Operator2/1 -> Select_05(1b)/1
  Lo`gical Operator3/1 -> Select_06(1b)/1
  Lo`gical Operator6/1 -> Select_04(1b)/1
  Lo`gical Operator19/1 -> Select_18(1b)/1
  Lo`gical Operator20/1 -> Select_19(1b)/1
  Lo`gical Operator21/1 -> Select_20(1b)/1
  Lo`gical Operator16/1 -> Select_16(1b)/1
  Lo`gical Operator24/1 -> Select_22(1b)/1
  Lo`gical Operator14/1 -> Select_03(1b)/1
  Lo`gical Operator25/1 -> Select_02(1b)/1
  Lo`gical Operator22/1 -> Select_01(1b)/1
  Lo`gical Operator31/1 -> Select_00(1b)/1

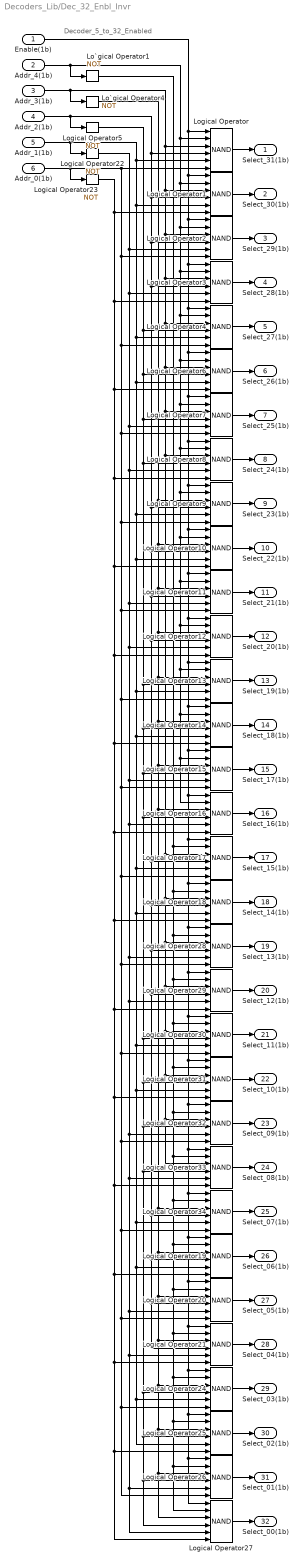
== system Decoders_Lib/Dec_32_Enbl_Invr ==
  note: Decoder_5_to_32_Enabled
  Enable(1b) : Inport
  Addr_4(1b) : Inport  Port=2
  Addr_3(1b) : Inport  Port=3
  Addr_2(1b) : Inport  Port=4
  Addr_1(1b) : Inport  Port=5
  Addr_0(1b) : Inport  Port=6
  Lo`gical Operator1 : Logic  Operator=NOT  IconShape=distinctive  AllPortsSameDT=off  OutDataTypeStr=boolean
  Lo`gical Operator4 : Logic  Operator=NOT  IconShape=distinctive  AllPortsSameDT=off  OutDataTypeStr=boolean
  Logical Operator{,1..4,6..21,24..34} (32 alike) : Logic  Operator=NAND  Inputs=6  IconShape=distinctive  AllPortsSameDT=off  OutDataTypeStr=boolean
  Logical Operator22 : Logic  Operator=NOT  IconShape=distinctive  AllPortsSameDT=off  OutDataTypeStr=boolean
  Logical Operator23 : Logic  Operator=NOT  IconShape=distinctive  AllPortsSameDT=off  OutDataTypeStr=boolean
  Logical Operator5 : Logic  Operator=NOT  IconShape=distinctive  AllPortsSameDT=off  OutDataTypeStr=boolean
  Select_31(1b) : Outport
  Select_30(1b) : Outport  Port=2
  Select_29(1b) : Outport  Port=3
  Select_28(1b) : Outport  Port=4
  Select_27(1b) : Outport  Port=5
  Select_26(1b) : Outport  Port=6
  Select_25(1b) : Outport  Port=7
  Select_24(1b) : Outport  Port=8
  Select_23(1b) : Outport  Port=9
  Select_22(1b) : Outport  Port=10
  Select_21(1b) : Outport  Port=11
  Select_20(1b) : Outport  Port=12
  Select_19(1b) : Outport  Port=13
  Select_18(1b) : Outport  Port=14
  Select_17(1b) : Outport  Port=15
  Select_16(1b) : Outport  Port=16
  Select_15(1b) : Outport  Port=17
  Select_14(1b) : Outport  Port=18
  Select_13(1b) : Outport  Port=19
  Select_12(1b) : Outport  Port=20
  Select_11(1b) : Outport  Port=21
  Select_10(1b) : Outport  Port=22
  Select_09(1b) : Outport  Port=23
  Select_08(1b) : Outport  Port=24
  Select_07(1b) : Outport  Port=25
  Select_06(1b) : Outport  Port=26
  Select_05(1b) : Outport  Port=27
  Select_04(1b) : Outport  Port=28
  Select_03(1b) : Outport  Port=29
  Select_02(1b) : Outport  Port=30
  Select_01(1b) : Outport  Port=31
  Select_00(1b) : Outport  Port=32
  wires:
  Logical Operator22/1 -> Logical Operator2/5, Logical Operator3/5, Logical Operator7/5, Logical Operator8/5, Logical Operator11/5, Logical Operator12/5, Logical Operator15/5, Logical Operator16/5, Logical Operator28/5, Logical Operator29/5, Logical Operator32/5, Logical Operator33/5, Logical Operator20/5, Logical Operator21/5, Logical Operator27/5, Logical Operator26/5
  Addr_0(1b)/1 -> Logical Operator2/6, Logical Operator4/6, Logical Operator7/6, Logical Operator9/6, Logical Operator11/6, Logical Operator13/6, Logical Operator15/6, Logical Operator17/6, Logical Operator28/6, Logical Operator30/6, Logical Operator32/6, Logical Operator34/6, Logical Operator20/6, Logical Operator24/6, Logical Operator26/6, Logical Operator/6, Logical Operator23/1
  Logical Operator23/1 -> Logical Operator1/6, Logical Operator3/6, Logical Operator6/6, Logical Operator8/6, Logical Operator10/6, Logical Operator12/6, Logical Operator14/6, Logical Operator16/6, Logical Operator18/6, Logical Operator29/6, Logical Operator31/6, Logical Operator33/6, Logical Operator19/6, Logical Operator21/6, Logical Operator27/6, Logical Operator25/6
  Logical Operator5/1 -> Logical Operator4/4, Logical Operator6/4, Logical Operator7/4, Logical Operator8/4, Logical Operator13/4, Logical Operator14/4, Logical Operator15/4, Logical Operator16/4, Logical Operator30/4, Logical Operator31/4, Logical Operator32/4, Logical Operator33/4, Logical Operator24/4, Logical Operator25/4, Logical Operator27/4, Logical Operator26/4
  Addr_3(1b)/1 -> Lo`gical Operator4/1, Logical Operator/3, Logical Operator1/3, Logical Operator2/3, Logical Operator3/3, Logical Operator4/3, Logical Operator6/3, Logical Operator7/3, Logical Operator8/3, Logical Operator17/3, Logical Operator18/3, Logical Operator28/3, Logical Operator29/3, Logical Operator30/3, Logical Operator31/3, Logical Operator33/3, Logical Operator32/3
  Addr_1(1b)/1 -> Logical Operator22/1, Logical Operator/5, Logical Operator1/5, Logical Operator4/5, Logical Operator6/5, Logical Operator9/5, Logical Operator10/5, Logical Operator13/5, Logical Operator14/5, Logical Operator17/5, Logical Operator18/5, Logical Operator30/5, Logical Operator31/5, Logical Operator34/5, Logical Operator19/5, Logical Operator24/5, Logical Operator25/5
  Addr_2(1b)/1 -> Logical Operator/4, Logical Operator1/4, Logical Operator2/4, Logical Operator3/4, Logical Operator9/4, Logical Operator10/4, Logical Operator11/4, Logical Operator12/4, Logical Operator17/4, Logical Operator18/4, Logical Operator28/4, Logical Operator29/4, Logical Operator34/4, Logical Operator19/4, Logical Operator21/4, Logical Operator20/4, Logical Operator5/1
  Lo`gical Operator4/1 -> Logical Operator9/3, Logical Operator10/3, Logical Operator11/3, Logical Operator12/3, Logical Operator13/3, Logical Operator14/3, Logical Operator15/3, Logical Operator16/3, Logical Operator34/3, Logical Operator19/3, Logical Operator20/3, Logical Operator21/3, Logical Operator24/3, Logical Operator25/3, Logical Operator26/3, Logical Operator27/3
  Lo`gical Operator1/1 -> Logical Operator17/2, Logical Operator18/2, Logical Operator28/2, Logical Operator29/2, Logical Operator30/2, Logical Operator31/2, Logical Operator32/2, Logical Operator33/2, Logical Operator34/2, Logical Operator19/2, Logical Operator20/2, Logical Operator21/2, Logical Operator24/2, Logical Operator25/2, Logical Operator26/2, Logical Operator27/2
  Addr_4(1b)/1 -> Logical Operator/2, Logical Operator1/2, Logical Operator2/2, Logical Operator3/2, Logical Operator4/2, Logical Operator6/2, Logical Operator7/2, Logical Operator8/2, Logical Operator9/2, Logical Operator10/2, Logical Operator11/2, Logical Operator12/2, Logical Operator13/2, Logical Operator14/2, Logical Operator15/2, Logical Operator16/2, Lo`gical Operator1/1
  Logical Operator3/1 -> Select_28(1b)/1
  Logical Operator4/1 -> Select_27(1b)/1
  Logical Operator7/1 -> Select_25(1b)/1
  Logical Operator16/1 -> Select_16(1b)/1
  Logical Operator8/1 -> Select_24(1b)/1
  Logical Operator15/1 -> Select_17(1b)/1
  Logical Operator14/1 -> Select_18(1b)/1
  Logical Operator11/1 -> Select_21(1b)/1
  Logical Operator12/1 -> Select_20(1b)/1
  Logical Operator9/1 -> Select_23(1b)/1
  Logical Operator34/1 -> Select_07(1b)/1
  Logical Operator30/1 -> Select_11(1b)/1
  Logical Operator10/1 -> Select_22(1b)/1
  Logical Operator31/1 -> Select_10(1b)/1
  Logical Operator/1 -> Select_31(1b)/1
  Logical Operator29/1 -> Select_12(1b)/1
  Logical Operator24/1 -> Select_03(1b)/1
  Logical Operator1/1 -> Select_30(1b)/1
  Logical Operator18/1 -> Select_14(1b)/1
  Logical Operator28/1 -> Select_13(1b)/1
  Logical Operator33/1 -> Select_08(1b)/1
  Logical Operator6/1 -> Select_26(1b)/1
  Logical Operator19/1 -> Select_06(1b)/1
  Logical Operator26/1 -> Select_01(1b)/1
  Logical Operator20/1 -> Select_05(1b)/1
  Logical Operator32/1 -> Select_09(1b)/1
  Logical Operator2/1 -> Select_29(1b)/1
  Logical Operator21/1 -> Select_04(1b)/1
  Logical Operator13/1 -> Select_19(1b)/1
  Logical Operator17/1 -> Select_15(1b)/1
  Logical Operator27/1 -> Select_00(1b)/1
  Logical Operator25/1 -> Select_02(1b)/1
  Enable(1b)/1 -> Logical Operator/1, Logical Operator1/1, Logical Operator2/1, Logical Operator3/1, Logical Operator4/1, Logical Operator6/1, Logical Operator7/1, Logical Operator8/1, Logical Operator9/1, Logical Operator10/1, Logical Operator11/1, Logical Operator12/1, Logical Operator13/1, Logical Operator14/1, Logical Operator15/1, Logical Operator16/1, Logical Operator17/1, Logical Operator18/1, Logical Operator28/1, Logical Operator29/1, Logical Operator30/1, Logical Operator31/1, Logical Operator32/1, Logical Operator33/1, Logical Operator34/1, Logical Operator19/1, Logical Operator20/1, Logical Operator21/1, Logical Operator24/1, Logical Operator25/1, Logical Operator26/1, Logical Operator27/1
